simulink model "VS_test"  (R2018a)
settings: Solver=FixedStepAuto  StartTime=0.0  StopTime=5  FixedStep=ST  RelTol=1e-3
undefined symbols (not defined in the file): delta, f, h, obj_points, theta_0, x_0, x_ref, y_0
settings Model: Creator=hkedw  LastModifiedBy=hkedw

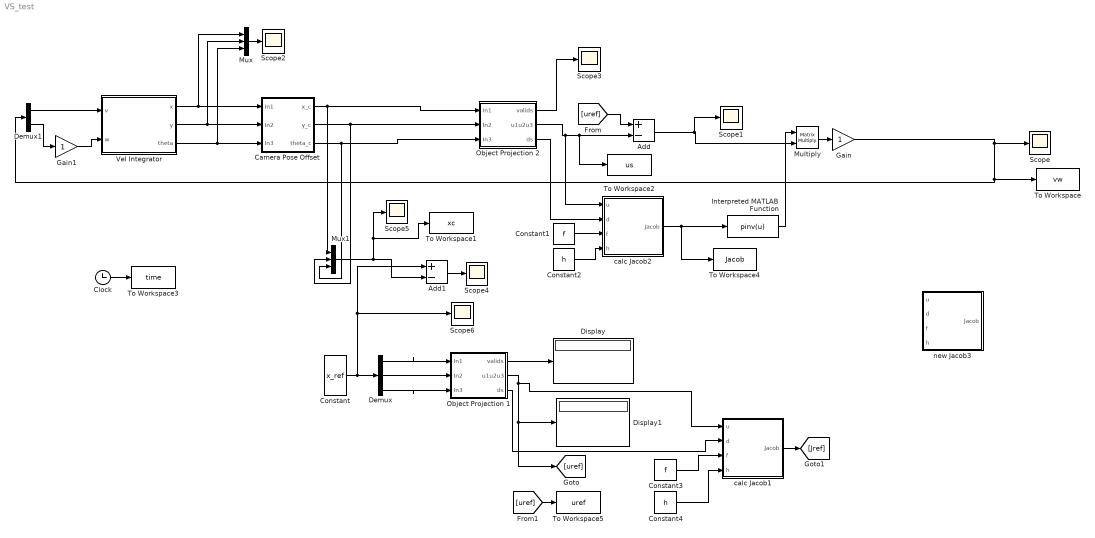
== system VS_test ==
  Add : Sum  Inputs=+-
  Add1 : Sum  Inputs=+-
  Camera Pose Offset : Subsystem
  Clock : Clock
  Constant : Constant  Value=x_ref  VectorParams1D=off
  Constant1 : Constant  Value=f
  Constant2 : Constant  Value=h
  Constant3 : Constant  Value=f
  Constant4 : Constant  Value=h
  Demux : Demux  Outputs=3
  Demux1 : Demux  Outputs=2
  Display : Display
  Display1 : Display
  Gain : Gain
  Gain1 : Gain
  Interpreted MATLAB Function : MATLABFcn  MATLABFcn=pinv(u)  Output1D=off
  Multiply : Product  Multiplication=Matrix(*)
  Mux : Mux  Inputs=3
  Mux1 : Mux  Inputs=3
  Object Projection 1 : Subsystem
  Object Projection 2 : Subsystem
  Scope{,1..6} (7 alike) : Scope
  To Workspace : ToWorkspace  VariableName=vw  SaveFormat=Timeseries  SampleTime=-1
  To Workspace1 : ToWorkspace  VariableName=xc  SaveFormat=Timeseries  SampleTime=-1
  To Workspace2 : ToWorkspace  VariableName=us  SaveFormat=Timeseries  SampleTime=-1
  To Workspace3 : ToWorkspace  VariableName=time  SaveFormat=Timeseries  SampleTime=-1
  To Workspace4 : ToWorkspace  VariableName=Jacob  SaveFormat=Timeseries  SampleTime=-1
  To Workspace5 : ToWorkspace  VariableName=uref  SaveFormat=Timeseries  SampleTime=-1
  Vel Integrator : Subsystem
  calc Jacob1 : MATLAB Function  TreatAsAtomicUnit=on
  calc Jacob2 : MATLAB Function  TreatAsAtomicUnit=on
  new Jacob3 : MATLAB Function  TreatAsAtomicUnit=on
  wires:
  Vel Integrator/1(x) -> Mux/1, Camera Pose Offset/1(In1)
  Vel Integrator/2(y) -> Mux/2, Camera Pose Offset/2(In2)
  Camera Pose Offset/1(x_c) -> Mux1/1, Object Projection 2/1(In1)
  Camera Pose Offset/2(y_c) -> Mux1/2, Object Projection 2/2(In2)
  Camera Pose Offset/3(theta_c) -> Mux1/3, Object Projection 2/3(In3)
  Object Projection 2/1(valids) -> Scope3/1
  Object Projection 2/2(u1u2u3) -> calc Jacob2/1(u), To Workspace2/1, Add/2
  Demux/1 -> Object Projection 1/1(In1)
  Demux/2 -> Object Projection 1/2(In2)
  Demux/3 -> Object Projection 1/3(In3)
  Object Projection 1/1(valids) -> Display/1
  Object Projection 1/2(u1u2u3) -> calc Jacob1/1(u), [uref], Display1/1
  [uref] -> Add/1
  Constant1/1 -> calc Jacob2/3(f)
  Constant2/1 -> calc Jacob2/4(h)
  Object Projection 1/3(ds) -> calc Jacob1/2(d)
  Constant3/1 -> calc Jacob1/3(f)
  Constant4/1 -> calc Jacob1/4(h)
  Interpreted MATLAB Function/1 -> Multiply/1
  Add/1 -> Multiply/2, Scope1/1
  Gain/1 -> To Workspace/1, Demux1/1, Scope/1
  Demux1/1 -> Vel Integrator/1(v)
  Gain1/1 -> Vel Integrator/2(w)
  Multiply/1 -> Gain/1
  Mux/1 -> Scope2/1
  Constant/1 -> Add1/1, Scope6/1, Demux/1
  Vel Integrator/3(theta) -> Mux/3, Camera Pose Offset/3(In3)
  Mux1/1 -> To Workspace1/1, Scope5/1, Add1/2
  Add1/1 -> Scope4/1
  Object Projection 2/3(ds) -> calc Jacob2/2(d)
  calc Jacob1/1(Jacob) -> [Jref]
  calc Jacob2/1(Jacob) -> To Workspace4/1, Interpreted MATLAB Function/1
  Clock/1 -> To Workspace3/1
  Demux1/2 -> Gain1/1
  [uref] -> To Workspace5/1

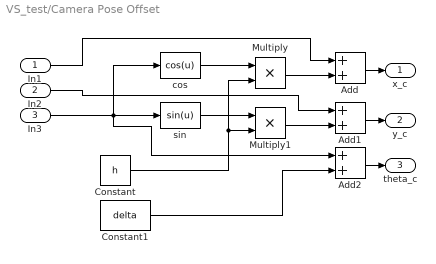
== system VS_test/Camera Pose Offset ==
  In1 : Inport
  In2 : Inport  Port=2
  In3 : Inport  Port=3
  Add : Sum
  Add1 : Sum
  Add2 : Sum
  Constant : Constant  Value=h
  Constant1 : Constant  Value=delta
  Multiply : Product
  Multiply1 : Product
  cos : MATLABFcn  MATLABFcn=cos(u)
  sin : MATLABFcn  MATLABFcn=sin(u)
  x_c : Outport
  y_c : Outport  Port=2
  theta_c : Outport  Port=3
  wires:
  Multiply/1 -> Add/2
  cos/1 -> Multiply/1
  In1/1 -> Add/1
  In3/1 -> Add2/1, cos/1, sin/1
  sin/1 -> Multiply1/1
  Constant1/1 -> Add2/2
  Multiply1/1 -> Add1/2
  Constant/1 -> Multiply1/2, Multiply/2
  In2/1 -> Add1/1
  Add1/1 -> y_c/1
  Add2/1 -> theta_c/1
  Add/1 -> x_c/1

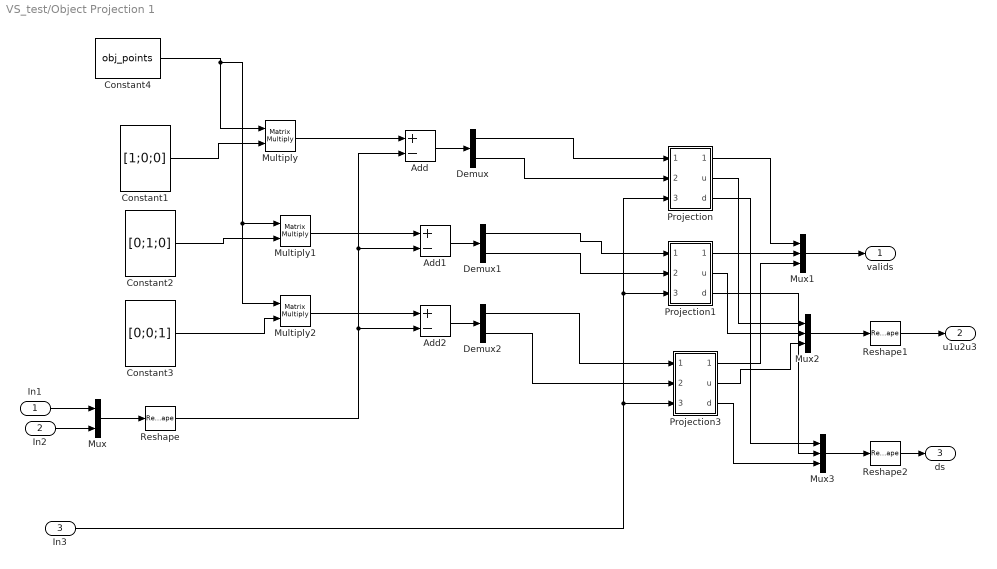
== system VS_test/Object Projection 1 ==
  In1 : Inport
  In2 : Inport  Port=2
  In3 : Inport  Port=3
  Add : Sum  Inputs=+-
  Add1 : Sum  Inputs=+-
  Add2 : Sum  Inputs=+-
  Constant1 : Constant  Value=[1;0;0]  VectorParams1D=off
  Constant2 : Constant  Value=[0;1;0]  VectorParams1D=off
  Constant3 : Constant  Value=[0;0;1]  VectorParams1D=off
  Constant4 : Constant  Value=obj_points
  Demux : Demux  Outputs=2
  Demux1 : Demux  Outputs=2
  Demux2 : Demux  Outputs=2
  Multiply : Product  Multiplication=Matrix(*)
  Multiply1 : Product  Multiplication=Matrix(*)
  Multiply2 : Product  Multiplication=Matrix(*)
  Mux : Mux  Inputs=2
  Mux1 : Mux  Inputs=3
  Mux2 : Mux  Inputs=3
  Mux3 : Mux  Inputs=3
  Projection : Subsystem
  Projection1 : Subsystem
  Projection3 : Subsystem
  Reshape : Reshape  OutputDimensionality=Column vector (2-D)
  Reshape1 : Reshape  OutputDimensionality=Column vector (2-D)
  Reshape2 : Reshape  OutputDimensionality=Column vector (2-D)
  valids : Outport
  u1u2u3 : Outport  Port=2
  ds : Outport  Port=3
  wires:
  Constant3/1 -> Multiply2/2
  Demux/2 -> Projection/2(In2)
  In3/1 -> Projection3/3(In3), Projection1/3(In3), Projection/3(In3)
  Constant2/1 -> Multiply1/2
  Demux1/1 -> Projection1/1(In1)
  Projection1/1(valid) -> Mux1/2
  Constant4/1 -> Multiply/1, Multiply2/1, Multiply1/1
  Constant1/1 -> Multiply/2
  Projection/1(valid) -> Mux1/1
  Mux1/1 -> valids/1
  Add1/1 -> Demux1/1
  Add2/1 -> Demux2/1
  Demux1/2 -> Projection1/2(In2)
  Multiply2/1 -> Add2/1
  Demux2/1 -> Projection3/1(In1)
  Multiply1/1 -> Add1/1
  Reshape/1 -> Add2/2, Add1/2, Add/2
  Projection3/1(valid) -> Mux1/3
  Projection1/2(u) -> Mux2/2
  Multiply/1 -> Add/1
  Projection/2(u) -> Mux2/1
  Demux2/2 -> Projection3/2(In2)
  Add/1 -> Demux/1
  Demux/1 -> Projection/1(In1)
  Projection3/2(u) -> Mux2/3
  In1/1 -> Mux/1
  In2/1 -> Mux/2
  Mux2/1 -> Reshape1/1
  Mux/1 -> Reshape/1
  Projection/3(d) -> Mux3/1
  Mux3/1 -> Reshape2/1
  Projection1/3(d) -> Mux3/2
  Projection3/3(d) -> Mux3/3
  Reshape1/1 -> u1u2u3/1
  Reshape2/1 -> ds/1

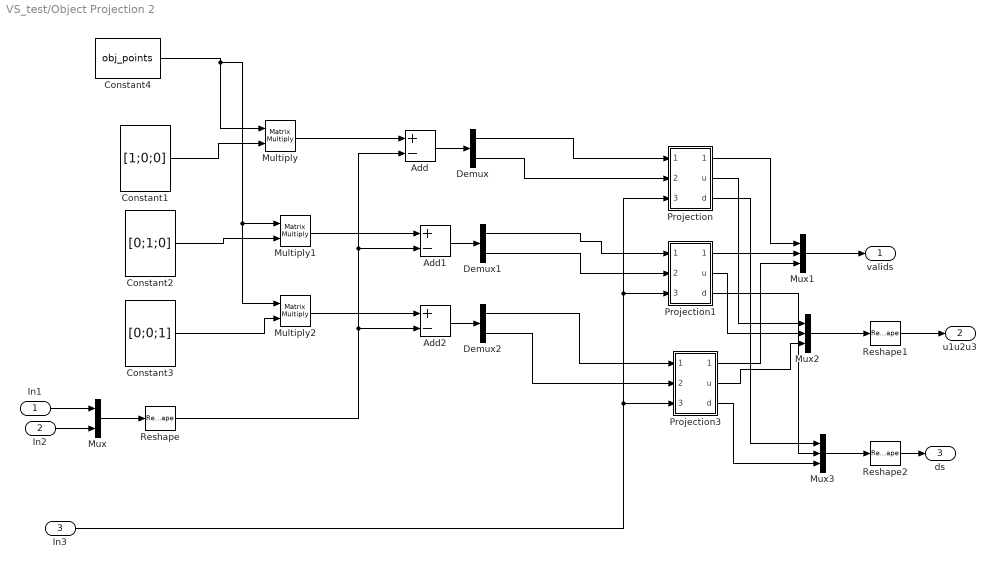
== system VS_test/Object Projection 2 ==
  In1 : Inport
  In2 : Inport  Port=2
  In3 : Inport  Port=3
  Add : Sum  Inputs=+-
  Add1 : Sum  Inputs=+-
  Add2 : Sum  Inputs=+-
  Constant1 : Constant  Value=[1;0;0]  VectorParams1D=off
  Constant2 : Constant  Value=[0;1;0]  VectorParams1D=off
  Constant3 : Constant  Value=[0;0;1]  VectorParams1D=off
  Constant4 : Constant  Value=obj_points
  Demux : Demux  Outputs=2
  Demux1 : Demux  Outputs=2
  Demux2 : Demux  Outputs=2
  Multiply : Product  Multiplication=Matrix(*)
  Multiply1 : Product  Multiplication=Matrix(*)
  Multiply2 : Product  Multiplication=Matrix(*)
  Mux : Mux  Inputs=2
  Mux1 : Mux  Inputs=3
  Mux2 : Mux  Inputs=3
  Mux3 : Mux  Inputs=3
  Projection : Subsystem
  Projection1 : Subsystem
  Projection3 : Subsystem
  Reshape : Reshape  OutputDimensionality=Column vector (2-D)
  Reshape1 : Reshape  OutputDimensionality=Column vector (2-D)
  Reshape2 : Reshape  OutputDimensionality=Column vector (2-D)
  valids : Outport
  u1u2u3 : Outport  Port=2
  ds : Outport  Port=3
  wires:
  Constant3/1 -> Multiply2/2
  Demux/2 -> Projection/2(In2)
  In3/1 -> Projection3/3(In3), Projection1/3(In3), Projection/3(In3)
  Constant2/1 -> Multiply1/2
  Demux1/1 -> Projection1/1(In1)
  Projection1/1(valid) -> Mux1/2
  Constant4/1 -> Multiply/1, Multiply2/1, Multiply1/1
  Constant1/1 -> Multiply/2
  Projection/1(valid) -> Mux1/1
  Mux1/1 -> valids/1
  Add1/1 -> Demux1/1
  Add2/1 -> Demux2/1
  Demux1/2 -> Projection1/2(In2)
  Multiply2/1 -> Add2/1
  Demux2/1 -> Projection3/1(In1)
  Multiply1/1 -> Add1/1
  Reshape/1 -> Add2/2, Add1/2, Add/2
  Projection3/1(valid) -> Mux1/3
  Projection1/2(u) -> Mux2/2
  Multiply/1 -> Add/1
  Projection/2(u) -> Mux2/1
  Demux2/2 -> Projection3/2(In2)
  Add/1 -> Demux/1
  Demux/1 -> Projection/1(In1)
  Projection3/2(u) -> Mux2/3
  In1/1 -> Mux/1
  In2/1 -> Mux/2
  Mux2/1 -> Reshape1/1
  Mux/1 -> Reshape/1
  Projection/3(d) -> Mux3/1
  Mux3/1 -> Reshape2/1
  Projection1/3(d) -> Mux3/2
  Projection3/3(d) -> Mux3/3
  Reshape1/1 -> u1u2u3/1
  Reshape2/1 -> ds/1

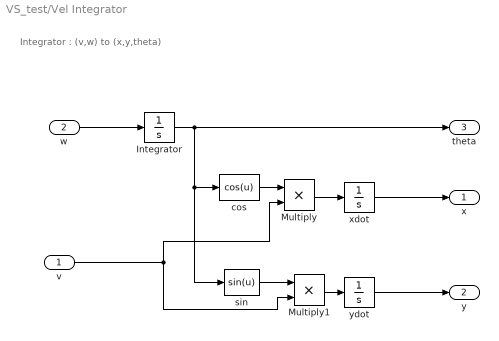
== system VS_test/Vel Integrator ==
  note: Integrator : (v,w) to (x,y,theta)
  v : Inport
  w : Inport  Port=2
  Integrator : Integrator  InitialCondition=theta_0
  Multiply : Product
  Multiply1 : Product
  cos : MATLABFcn  MATLABFcn=cos(u)
  sin : MATLABFcn  MATLABFcn=sin(u)
  xdot : Integrator  InitialCondition=x_0
  ydot : Integrator  InitialCondition=y_0
  x : Outport
  y : Outport  Port=2
  theta : Outport  Port=3
  wires:
  w/1 -> Integrator/1
  Multiply/1 -> xdot/1
  cos/1 -> Multiply/1
  Multiply1/1 -> ydot/1
  ydot/1 -> y/1
  xdot/1 -> x/1
  sin/1 -> Multiply1/1
  Integrator/1 -> theta/1, sin/1, cos/1
  v/1 -> Multiply/2, Multiply1/2

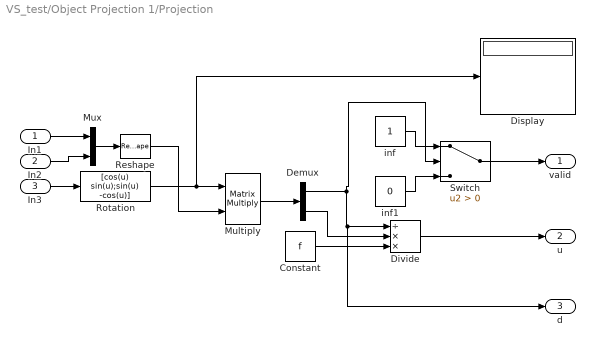
== system VS_test/Object Projection 1/Projection ==
  In1 : Inport
  In2 : Inport  Port=2
  In3 : Inport  Port=3
  Constant : Constant  Value=f
  Demux : Demux  Outputs=2
  Display : Display
  Divide : Product  Inputs=/**
  Multiply : Product  Multiplication=Matrix(*)
  Mux : Mux  Inputs=2
  Reshape : Reshape  OutputDimensionality=Column vector (2-D)
  Rotation : MATLABFcn  MATLABFcn=[cos(u) sin(u);sin(u) -cos(u)]  OutputDimensions=[2 2]  Output1D=off
  Switch : Switch  Criteria=u2 > Threshold
  inf : Constant
  inf1 : Constant  Value=0
  valid : Outport
  u : Outport  Port=2
  d : Outport  Port=3
  wires:
  Demux/2 -> Divide/2
  Switch/1 -> valid/1
  Demux/1 -> Switch/2, d/1, Divide/1
  Constant/1 -> Divide/3
  Mux/1 -> Reshape/1
  Reshape/1 -> Multiply/2
  In2/1 -> Mux/2
  Multiply/1 -> Demux/1
  inf/1 -> Switch/1
  inf1/1 -> Switch/3
  In3/1 -> Rotation/1
  In1/1 -> Mux/1
  Divide/1 -> u/1
  Rotation/1 -> Display/1, Multiply/1

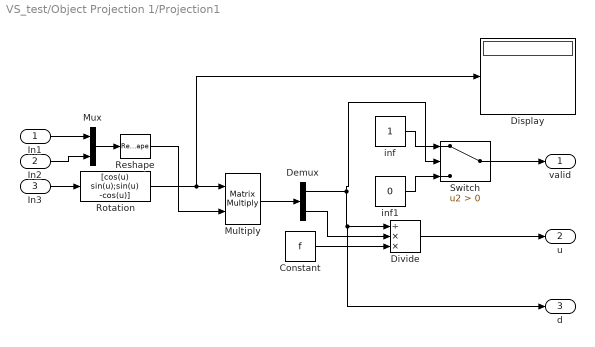
== system VS_test/Object Projection 1/Projection1 ==
  In1 : Inport
  In2 : Inport  Port=2
  In3 : Inport  Port=3
  Constant : Constant  Value=f
  Demux : Demux  Outputs=2
  Display : Display
  Divide : Product  Inputs=/**
  Multiply : Product  Multiplication=Matrix(*)
  Mux : Mux  Inputs=2
  Reshape : Reshape  OutputDimensionality=Column vector (2-D)
  Rotation : MATLABFcn  MATLABFcn=[cos(u) sin(u);sin(u) -cos(u)]  OutputDimensions=[2 2]  Output1D=off
  Switch : Switch  Criteria=u2 > Threshold
  inf : Constant
  inf1 : Constant  Value=0
  valid : Outport
  u : Outport  Port=2
  d : Outport  Port=3
  wires:
  Demux/2 -> Divide/2
  Switch/1 -> valid/1
  Demux/1 -> Switch/2, d/1, Divide/1
  Constant/1 -> Divide/3
  Mux/1 -> Reshape/1
  Reshape/1 -> Multiply/2
  In2/1 -> Mux/2
  Multiply/1 -> Demux/1
  inf/1 -> Switch/1
  inf1/1 -> Switch/3
  In3/1 -> Rotation/1
  In1/1 -> Mux/1
  Divide/1 -> u/1
  Rotation/1 -> Display/1, Multiply/1

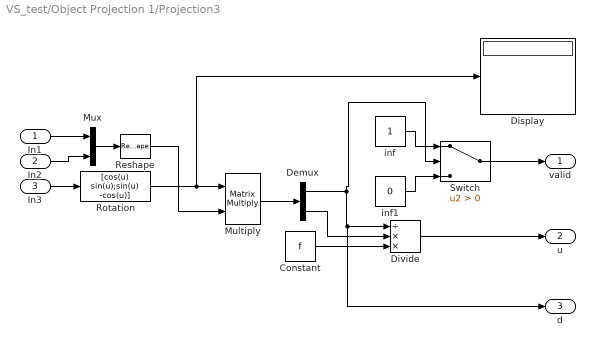
== system VS_test/Object Projection 1/Projection3 ==
  In1 : Inport
  In2 : Inport  Port=2
  In3 : Inport  Port=3
  Constant : Constant  Value=f
  Demux : Demux  Outputs=2
  Display : Display
  Divide : Product  Inputs=/**
  Multiply : Product  Multiplication=Matrix(*)
  Mux : Mux  Inputs=2
  Reshape : Reshape  OutputDimensionality=Column vector (2-D)
  Rotation : MATLABFcn  MATLABFcn=[cos(u) sin(u);sin(u) -cos(u)]  OutputDimensions=[2 2]  Output1D=off
  Switch : Switch  Criteria=u2 > Threshold
  inf : Constant
  inf1 : Constant  Value=0
  valid : Outport
  u : Outport  Port=2
  d : Outport  Port=3
  wires:
  Demux/2 -> Divide/2
  Switch/1 -> valid/1
  Demux/1 -> Switch/2, d/1, Divide/1
  Constant/1 -> Divide/3
  Mux/1 -> Reshape/1
  Reshape/1 -> Multiply/2
  In2/1 -> Mux/2
  Multiply/1 -> Demux/1
  inf/1 -> Switch/1
  inf1/1 -> Switch/3
  In3/1 -> Rotation/1
  In1/1 -> Mux/1
  Divide/1 -> u/1
  Rotation/1 -> Display/1, Multiply/1

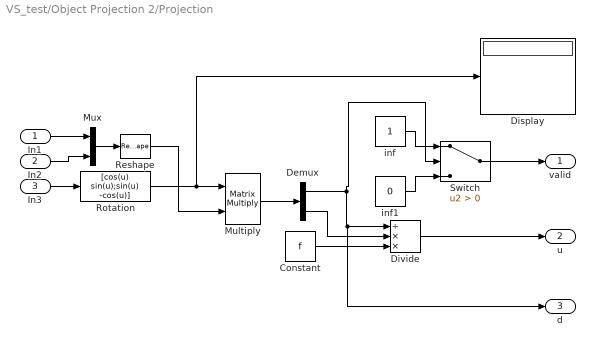
== system VS_test/Object Projection 2/Projection ==
  In1 : Inport
  In2 : Inport  Port=2
  In3 : Inport  Port=3
  Constant : Constant  Value=f
  Demux : Demux  Outputs=2
  Display : Display
  Divide : Product  Inputs=/**
  Multiply : Product  Multiplication=Matrix(*)
  Mux : Mux  Inputs=2
  Reshape : Reshape  OutputDimensionality=Column vector (2-D)
  Rotation : MATLABFcn  MATLABFcn=[cos(u) sin(u);sin(u) -cos(u)]  OutputDimensions=[2 2]  Output1D=off
  Switch : Switch  Criteria=u2 > Threshold
  inf : Constant
  inf1 : Constant  Value=0
  valid : Outport
  u : Outport  Port=2
  d : Outport  Port=3
  wires:
  Demux/2 -> Divide/2
  Switch/1 -> valid/1
  Demux/1 -> Switch/2, d/1, Divide/1
  Constant/1 -> Divide/3
  Mux/1 -> Reshape/1
  Reshape/1 -> Multiply/2
  In2/1 -> Mux/2
  Multiply/1 -> Demux/1
  inf/1 -> Switch/1
  inf1/1 -> Switch/3
  In3/1 -> Rotation/1
  In1/1 -> Mux/1
  Divide/1 -> u/1
  Rotation/1 -> Display/1, Multiply/1

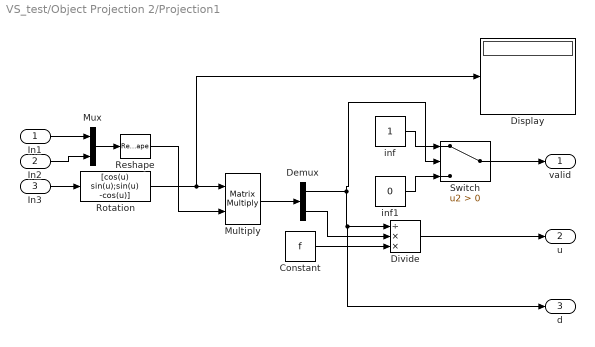
== system VS_test/Object Projection 2/Projection1 ==
  In1 : Inport
  In2 : Inport  Port=2
  In3 : Inport  Port=3
  Constant : Constant  Value=f
  Demux : Demux  Outputs=2
  Display : Display
  Divide : Product  Inputs=/**
  Multiply : Product  Multiplication=Matrix(*)
  Mux : Mux  Inputs=2
  Reshape : Reshape  OutputDimensionality=Column vector (2-D)
  Rotation : MATLABFcn  MATLABFcn=[cos(u) sin(u);sin(u) -cos(u)]  OutputDimensions=[2 2]  Output1D=off
  Switch : Switch  Criteria=u2 > Threshold
  inf : Constant
  inf1 : Constant  Value=0
  valid : Outport
  u : Outport  Port=2
  d : Outport  Port=3
  wires:
  Demux/2 -> Divide/2
  Switch/1 -> valid/1
  Demux/1 -> Switch/2, d/1, Divide/1
  Constant/1 -> Divide/3
  Mux/1 -> Reshape/1
  Reshape/1 -> Multiply/2
  In2/1 -> Mux/2
  Multiply/1 -> Demux/1
  inf/1 -> Switch/1
  inf1/1 -> Switch/3
  In3/1 -> Rotation/1
  In1/1 -> Mux/1
  Divide/1 -> u/1
  Rotation/1 -> Display/1, Multiply/1

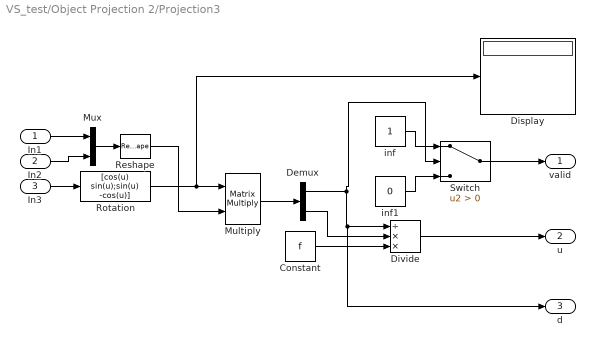
== system VS_test/Object Projection 2/Projection3 ==
  In1 : Inport
  In2 : Inport  Port=2
  In3 : Inport  Port=3
  Constant : Constant  Value=f
  Demux : Demux  Outputs=2
  Display : Display
  Divide : Product  Inputs=/**
  Multiply : Product  Multiplication=Matrix(*)
  Mux : Mux  Inputs=2
  Reshape : Reshape  OutputDimensionality=Column vector (2-D)
  Rotation : MATLABFcn  MATLABFcn=[cos(u) sin(u);sin(u) -cos(u)]  OutputDimensions=[2 2]  Output1D=off
  Switch : Switch  Criteria=u2 > Threshold
  inf : Constant
  inf1 : Constant  Value=0
  valid : Outport
  u : Outport  Port=2
  d : Outport  Port=3
  wires:
  Demux/2 -> Divide/2
  Switch/1 -> valid/1
  Demux/1 -> Switch/2, d/1, Divide/1
  Constant/1 -> Divide/3
  Mux/1 -> Reshape/1
  Reshape/1 -> Multiply/2
  In2/1 -> Mux/2
  Multiply/1 -> Demux/1
  inf/1 -> Switch/1
  inf1/1 -> Switch/3
  In3/1 -> Rotation/1
  In1/1 -> Mux/1
  Divide/1 -> u/1
  Rotation/1 -> Display/1, Multiply/1

== matlab function VS_test/calc Jacob1 ==
  data: u input; Jacob output; d input; f input; h input
function Jacob = fcn(u,d,f,h)

u = reshape(u,3,1);
d = reshape(d,3,1);

Jacob = [u 1./d*h*f+f-d.*u.*u/f]

== matlab function VS_test/new Jacob3 ==
  data: u input; Jacob output; d input; f input; h input
function Jacob  = fcn(u,d,f,h)

u = reshape(u,3,1);
d = reshape(d,3,1);

Jacob = [u 1./f+f*h./d-u.*u/f]

== matlab function VS_test/calc Jacob2 ==
  data: u input; Jacob output; d input; f input; h input
function Jacob  = fcn(u,d,f,h)

u = reshape(u,3,1);
d = reshape(d,3,1);

Jacob = [u 1./f+f*h./d-u.*u/f]
